simulink library "GearLibrary"  (R2017b)
settings: Solver=VariableStepAuto  StartTime=0.0  StopTime=10.0  RelTol=1e-3
undefined symbols (not defined in the file): c_LTset, DiscIntNeverNeededParam, g, Gear, magnitude, Strut, Tss, x1_LTset
libraries: GearLibrary x11, BaseLibrary x6, simulink x4, MathLibrary x2, vrlib x1
(part 2 of 2)

== system GearLibrary/Forces in Contact Point_Z2/If Action Subsystem1 ==
  v : Inport
  x : Inport  Port=2
  Action Port : ActionPort  InitializeStates=reset  ActionType=elseif
  " " : Saturate  UpperLimit=FOR_MaxDamp  LowerLimit=-FOR_MaxDamp
  Add : Sum
  Gain7 : Gain  Gain=d
  Gain8 : Gain  Gain=c
  Saturation : Saturate  UpperLimit=Compress_LengthMax*c  LowerLimit=-Compress_LengthMax*c
  Fz : Outport
  wires:
  v/1 -> Gain7/1  "x1dot"
  x/1 -> Gain8/1  "x1"
  Gain8/1 -> Saturation/1
  Add/1 -> Fz/1  "Fz1"
  Saturation/1 -> Add/2  "Fc"
  Gain7/1 -> " "/1
  " "/1 -> Add/1  "Fd"

== system GearLibrary/Forces in Contact Point_Z2/If Action Subsystem2 ==
  v : Inport
  x : Inport  Port=2
  Action Port : ActionPort  InitializeStates=reset  ActionType=else
  Add : Sum
  Constant : Constant  Value=Compress_LengthMax
  Constant1 : Constant  Value=Compress_LengthMax*c
  Fc2tox2 : Lookup_n-D  NumberOfTableDimensions=1  BreakpointsForDimension1=(linspace(0,Compress_LengthMax_Tire,30) * (9 * ct / Compress_LengthMax_Tire) + ct).*linspace(0,Compress_LengthMax_Tire,30)  Table=linspace(0,Compress_LengthMax_Tire,30)  InternalRulePriority=Speed  RndMeth=Simplest  InputSameDT=on
  Gain : Gain  Gain=-1
  Gain1 : Gain  Gain=-1
  Gain12 : Gain  Gain=dt
  Saturation : Saturate  UpperLimit=0  LowerLimit=-10*ct*Compress_LengthMax_Tire
  Sum : Sum  Inputs=|++
  Sum1 : Sum  Inputs=|+-
  x2toFc2 : Lookup_n-D  NumberOfTableDimensions=1  BreakpointsForDimension1=linspace(0,Compress_LengthMax_Tire,30)  Table=(linspace(0,Compress_LengthMax_Tire,30) * (9 * ct / Compress_LengthMax_Tire) + ct).*linspace(0,Compress_LengthMax_Tire,30)  InternalRulePriority=Speed  RndMeth=Simplest  InputSameDT=on
  Fz : Outport
  wires:
  x/1 -> Sum/1
  v/1 -> Gain12/1
  Sum/1 -> Sum1/1
  Constant/1 -> Sum/2
  x2toFc2/1 -> Gain1/1
  Gain12/1 -> Add/1  "Fdt"
  Saturation/1 -> Add/2  "Fct"
  Add/1 -> Fz/1  "Fz2"
  Constant1/1 -> Fc2tox2/1
  Sum1/1 -> Gain/1
  Gain/1 -> x2toFc2/1
  Gain1/1 -> Saturation/1
  Fc2tox2/1 -> Sum1/2

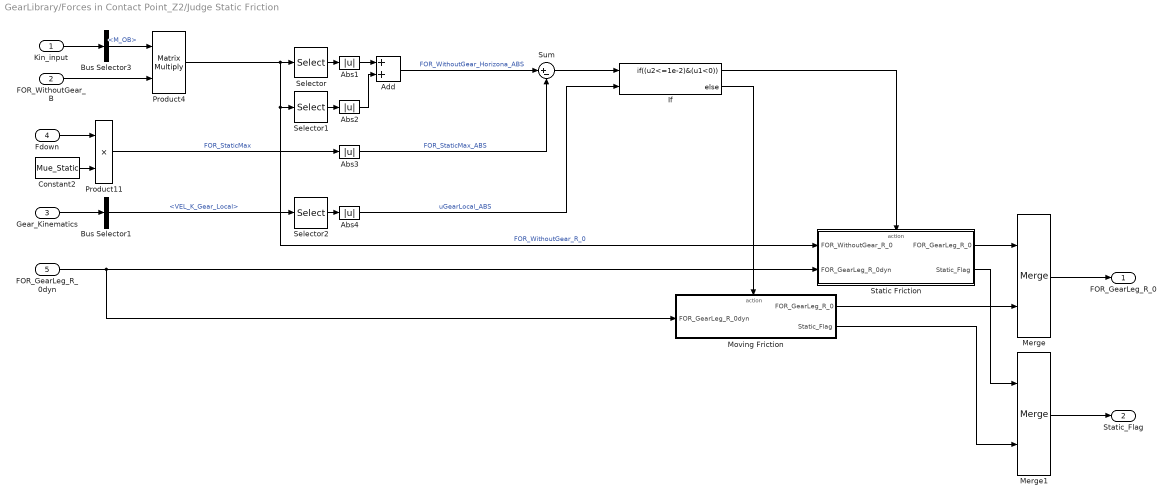
== system GearLibrary/Forces in Contact Point_Z2/Judge Static Friction ==
  Kin_input : Inport  OutDataTypeStr=Bus: Kin_input_BUS
  FOR_WithoutGear_B : Inport  Port=2  Unit=N  PortDimensions=[3 1]
  Gear_Kinematics : Inport  Port=3  OutDataTypeStr=Bus: GearKinematics_BUS
  Fdown : Inport  Port=4
  FOR_GearLeg_R_0dyn : Inport  Port=5
  Abs{1..4} (4 alike) : Abs
  Add : Sum
  Bus Selector1 : BusSelector  OutputSignals=VEL_K_Gear_Local
  Bus Selector3 : BusSelector  OutputSignals=M_OB
  Constant2 : Constant  Value=Mue_Static
  If : If  NumInputs=2  IfExpression=(u2<=1e-2)&(u1<0)
  Merge : Merge
  Merge1 : Merge
  Moving Friction : Subsystem  TreatAsAtomicUnit=on
  Product11 : Product
  Product4 : Product  Multiplication=Matrix(*)
  Selector : Selector  InputPortWidth=3  IndexOptions=Index vector (dialog)  Indices=[1]  OutputSizes=1
  Selector1 : Selector  InputPortWidth=3  IndexOptions=Index vector (dialog)  Indices=[2]  OutputSizes=1
  Selector2 : Selector  InputPortWidth=3  IndexOptions=Index vector (dialog)  Indices=[1]  OutputSizes=1
  "Static Friction " : Subsystem  TreatAsAtomicUnit=on
  Sum : Sum  Inputs=|+-
  FOR_GearLeg_R_0 : Outport  Unit=N  PortDimensions=[3,1]
  Static_Flag : Outport  Port=2  PortDimensions=[1]
  wires:
  "Static Friction "/2(Static_Flag) -> Merge1/1
  Merge1/1 -> Static_Flag/1
  Moving Friction/2(Static_Flag) -> Merge1/2
  Merge/1 -> FOR_GearLeg_R_0/1
  Moving Friction/1(FOR_GearLeg_R_0) -> Merge/2
  FOR_GearLeg_R_0dyn/1 -> Moving Friction/1(FOR_GearLeg_R_0dyn), "Static Friction "/2(FOR_GearLeg_R_0dyn)
  If/2 -> Moving Friction/Action
  "Static Friction "/1(FOR_GearLeg_R_0) -> Merge/1
  If/1 -> "Static Friction "/Action
  Abs4/1 -> If/2  "uGearLocal_ABS"
  Selector2/1 -> Abs4/1
  Bus Selector1/1 -> Selector2/1  "<VEL_K_Gear_Local>"
  Gear_Kinematics/1 -> Bus Selector1/1
  Sum/1 -> If/1
  Abs3/1 -> Sum/2  "FOR_StaticMax_ABS"
  Abs2/1 -> Add/2
  Selector1/1 -> Abs2/1
  Selector/1 -> Abs1/1
  Abs1/1 -> Add/1
  Add/1 -> Sum/1  "FOR_WithoutGear_Horizona_ABS"
  Product4/1 -> Selector/1, Selector1/1, "Static Friction "/1(FOR_WithoutGear_R_0)  "FOR_WithoutGear_R_0"
  FOR_WithoutGear_B/1 -> Product4/2
  Bus Selector3/1 -> Product4/1  "<M_OB>"
  Kin_input/1 -> Bus Selector3/1
  Product11/1 -> Abs3/1  "FOR_StaticMax"
  Constant2/1 -> Product11/2
  Fdown/1 -> Product11/1

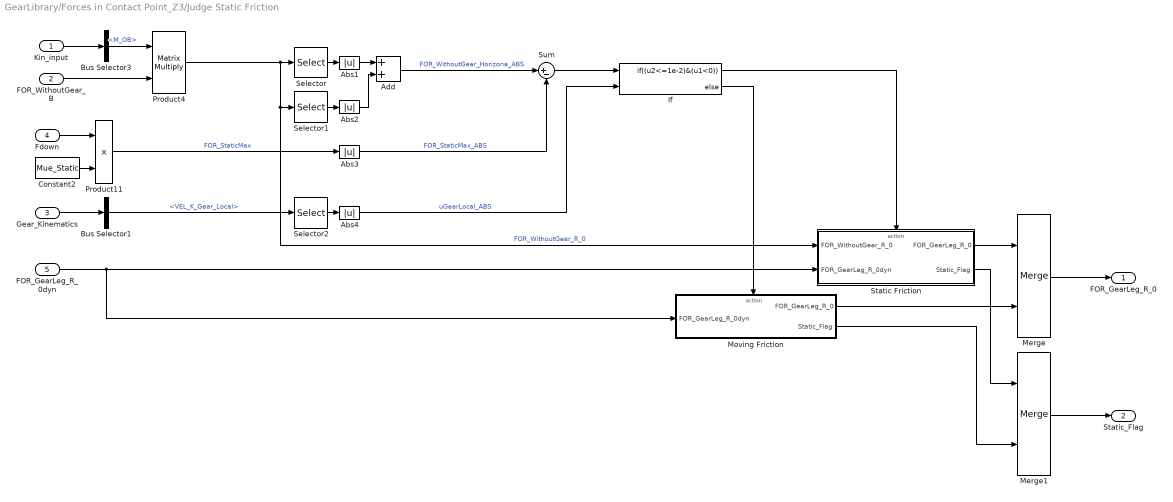
== system GearLibrary/Forces in Contact Point_Z3/Judge Static Friction ==
  Kin_input : Inport  OutDataTypeStr=Bus: Kin_input_BUS
  FOR_WithoutGear_B : Inport  Port=2  Unit=N  PortDimensions=[3 1]
  Gear_Kinematics : Inport  Port=3  OutDataTypeStr=Bus: GearKinematics_BUS
  Fdown : Inport  Port=4
  FOR_GearLeg_R_0dyn : Inport  Port=5
  Abs{1..4} (4 alike) : Abs
  Add : Sum
  Bus Selector1 : BusSelector  OutputSignals=VEL_K_Gear_Local
  Bus Selector3 : BusSelector  OutputSignals=M_OB
  Constant2 : Constant  Value=Mue_Static  SampleTime=Tss
  If : If  NumInputs=2  IfExpression=(u2<=1e-2)&(u1<0)
  Merge : Merge
  Merge1 : Merge
  Moving Friction : Subsystem  TreatAsAtomicUnit=on
  Product11 : Product
  Product4 : Product  Multiplication=Matrix(*)
  Selector : Selector  InputPortWidth=3  IndexOptions=Index vector (dialog)  Indices=[1]  OutputSizes=1
  Selector1 : Selector  InputPortWidth=3  IndexOptions=Index vector (dialog)  Indices=[2]  OutputSizes=1
  Selector2 : Selector  InputPortWidth=3  IndexOptions=Index vector (dialog)  Indices=[1]  OutputSizes=1
  "Static Friction " : Subsystem  TreatAsAtomicUnit=on
  Sum : Sum  Inputs=|+-
  FOR_GearLeg_R_0 : Outport  Unit=N  PortDimensions=[3,1]
  Static_Flag : Outport  Port=2  PortDimensions=[1]
  wires:
  "Static Friction "/2(Static_Flag) -> Merge1/1
  Merge1/1 -> Static_Flag/1
  Moving Friction/2(Static_Flag) -> Merge1/2
  Merge/1 -> FOR_GearLeg_R_0/1
  Moving Friction/1(FOR_GearLeg_R_0) -> Merge/2
  FOR_GearLeg_R_0dyn/1 -> Moving Friction/1(FOR_GearLeg_R_0dyn), "Static Friction "/2(FOR_GearLeg_R_0dyn)
  If/2 -> Moving Friction/Action
  "Static Friction "/1(FOR_GearLeg_R_0) -> Merge/1
  If/1 -> "Static Friction "/Action
  Abs4/1 -> If/2  "uGearLocal_ABS"
  Selector2/1 -> Abs4/1
  Bus Selector1/1 -> Selector2/1  "<VEL_K_Gear_Local>"
  Gear_Kinematics/1 -> Bus Selector1/1
  Sum/1 -> If/1
  Abs3/1 -> Sum/2  "FOR_StaticMax_ABS"
  Abs2/1 -> Add/2
  Selector1/1 -> Abs2/1
  Selector/1 -> Abs1/1
  Abs1/1 -> Add/1
  Add/1 -> Sum/1  "FOR_WithoutGear_Horizona_ABS"
  Product4/1 -> Selector/1, Selector1/1, "Static Friction "/1(FOR_WithoutGear_R_0)  "FOR_WithoutGear_R_0"
  FOR_WithoutGear_B/1 -> Product4/2
  Bus Selector3/1 -> Product4/1  "<M_OB>"
  Kin_input/1 -> Bus Selector3/1
  Product11/1 -> Abs3/1  "FOR_StaticMax"
  Constant2/1 -> Product11/2
  Fdown/1 -> Product11/1

== system GearLibrary/Gear Contact Point Dynamics/Calc VEL local lon//lat ==
  VEL_K_Gear_NED : Inport
  Tire Heading : Inport  Port=2  Unit=rad  PortDimensions=[1,1]
  Add : Sum
  Add1 : Sum
  Cos : Trigonometry  Operator=cos
  Cos1 : Trigonometry
  Cos2 : Trigonometry
  Cos3 : Trigonometry  Operator=cos
  Gain : Gain  Gain=-1
  Product{,1..3} (4 alike) : Product
  Vector Concatenate : Concatenate  NumInputs=3  Mode=Multidimensional array
  uB : Selector  InputPortWidth=3  IndexOptions=Index vector (dialog)  Indices=[1]  OutputSizes=1
  "uB " : Selector  InputPortWidth=3  IndexOptions=Index vector (dialog)  Indices=[1]  OutputSizes=1
  vB : Selector  InputPortWidth=3  IndexOptions=Index vector (dialog)  Indices=[2]  OutputSizes=1
  "vB " : Selector  InputPortWidth=3  IndexOptions=Index vector (dialog)  Indices=[2]  OutputSizes=1
  wB : Selector  InputPortWidth=3  IndexOptions=Index vector (dialog)  Indices=[3]  OutputSizes=1
  VEL_K_Gear_Local : Outport  Unit=m/s  PortDimensions=[3 1]
  wires:
  Tire Heading/1 -> Cos2/1, Cos3/1, Cos1/1, Cos/1
  VEL_K_Gear_NED/1 -> wB/1, "vB "/1, "uB "/1, vB/1, uB/1
  Cos/1 -> Product/1
  Product/1 -> Add/1
  uB/1 -> Product/2
  vB/1 -> Product1/2
  Cos1/1 -> Product1/1
  Product1/1 -> Add/2
  Add/1 -> Vector Concatenate/1
  Vector Concatenate/1 -> VEL_K_Gear_Local/1
  "uB "/1 -> Gain/1
  Gain/1 -> Product2/2
  Cos2/1 -> Product2/1
  "vB "/1 -> Product3/2
  Cos3/1 -> Product3/1
  Product3/1 -> Add1/2
  Product2/1 -> Add1/1
  Add1/1 -> Vector Concatenate/2
  wB/1 -> Vector Concatenate/3

== system GearLibrary/Gear Contact Point Dynamics/Norm ==
  V : Inport
  Math Function : Math  Operator=magnitude^2  SaturateOnIntegerOverflow=on
  Sqrt : Sqrt  SaturateOnIntegerOverflow=on
  Sum4 : Sum  Inputs=+
  ||V|| : Outport
  wires:
  Math Function/1 -> Sum4/1
  Sum4/1 -> Sqrt/1
  Sqrt/1 -> ||V||/1
  V/1 -> Math Function/1

== system GearLibrary/Gear Contact Point Dynamics/Subsystem ==
  Angle : Inport
  Trigonometric Function : Trigonometry  Operator=sincos
  Trigonometric Function1 : Trigonometry  Operator=atan2
  AngleWrap : Outport
  wires:
  Angle/1 -> Trigonometric Function/1
  Trigonometric Function/1 -> Trigonometric Function1/1
  Trigonometric Function/2 -> Trigonometric Function1/2
  Trigonometric Function1/1 -> AngleWrap/1

== system GearLibrary/Gear Contact Point Dynamics_WL1/Calc VEL local lon//lat ==
  VEL_K_Gear_NED : Inport
  Tire Heading : Inport  Port=2  Unit=rad  PortDimensions=[1,1]
  Add : Sum
  Add1 : Sum
  Cos : Trigonometry  Operator=cos
  Cos1 : Trigonometry
  Cos2 : Trigonometry
  Cos3 : Trigonometry  Operator=cos
  Gain : Gain  Gain=-1
  Product{,1..3} (4 alike) : Product
  Vector Concatenate : Concatenate  NumInputs=3  Mode=Multidimensional array
  uB : Selector  InputPortWidth=3  IndexOptions=Index vector (dialog)  Indices=[1]  OutputSizes=1
  "uB " : Selector  InputPortWidth=3  IndexOptions=Index vector (dialog)  Indices=[1]  OutputSizes=1
  vB : Selector  InputPortWidth=3  IndexOptions=Index vector (dialog)  Indices=[2]  OutputSizes=1
  "vB " : Selector  InputPortWidth=3  IndexOptions=Index vector (dialog)  Indices=[2]  OutputSizes=1
  wB : Selector  InputPortWidth=3  IndexOptions=Index vector (dialog)  Indices=[3]  OutputSizes=1
  VEL_K_Gear_Local : Outport  Unit=m/s  PortDimensions=[3 1]
  wires:
  wB/1 -> Vector Concatenate/3
  Add1/1 -> Vector Concatenate/2
  Product2/1 -> Add1/1
  Product3/1 -> Add1/2
  Cos3/1 -> Product3/1
  "vB "/1 -> Product3/2
  Cos2/1 -> Product2/1
  Gain/1 -> Product2/2
  "uB "/1 -> Gain/1
  Vector Concatenate/1 -> VEL_K_Gear_Local/1
  Add/1 -> Vector Concatenate/1
  Product1/1 -> Add/2
  Cos1/1 -> Product1/1
  vB/1 -> Product1/2
  uB/1 -> Product/2
  Product/1 -> Add/1
  Cos/1 -> Product/1
  VEL_K_Gear_NED/1 -> uB/1, vB/1, "uB "/1, "vB "/1, wB/1
  Tire Heading/1 -> Cos/1, Cos1/1, Cos3/1, Cos2/1

== system GearLibrary/Gear Contact Point Dynamics_WL1/Norm ==
  V : Inport
  Math Function : Math  Operator=magnitude^2  SaturateOnIntegerOverflow=on
  Sqrt : Sqrt  SaturateOnIntegerOverflow=on
  Sum4 : Sum  Inputs=+
  ||V|| : Outport
  wires:
  V/1 -> Math Function/1
  Sqrt/1 -> ||V||/1
  Sum4/1 -> Sqrt/1
  Math Function/1 -> Sum4/1

== system GearLibrary/Gear Contact Point Dynamics_WL1/Subsystem ==
  Angle : Inport
  Trigonometric Function : Trigonometry  Operator=sincos
  Trigonometric Function1 : Trigonometry  Operator=atan2
  AngleWrap : Outport
  wires:
  Trigonometric Function1/1 -> AngleWrap/1
  Trigonometric Function/2 -> Trigonometric Function1/2
  Trigonometric Function/1 -> Trigonometric Function1/1
  Angle/1 -> Trigonometric Function/1

== system GearLibrary/Forces in Contact Point/Judge Static Friction/Moving Friction ==
  FOR_GearLeg_R_0dyn : Inport
  Action Port : ActionPort  ActionType=else
  Constant : Constant  Value=0
  FOR_GearLeg_R_0 : Outport  Unit=N  PortDimensions=[3,1]
  Static_Flag : Outport  Port=2  PortDimensions=[1]
  wires:
  FOR_GearLeg_R_0dyn/1 -> FOR_GearLeg_R_0/1
  Constant/1 -> Static_Flag/1

== system GearLibrary/Forces in Contact Point/Judge Static Friction/Static Friction  ==
  FOR_WithoutGear_R_0 : Inport
  FOR_GearLeg_R_0dyn : Inport  Port=2
  Action Port : ActionPort  ActionType=then
  Constant : Constant
  Selector : Selector  InputPortWidth=3  IndexOptions=Index vector (dialog)  Indices=[1]  OutputSizes=1
  Selector1 : Selector  InputPortWidth=3  IndexOptions=Index vector (dialog)  Indices=[2]  OutputSizes=1
  Selector2 : Selector  InputPortWidth=3  IndexOptions=Index vector (dialog)  Indices=[3]  OutputSizes=1
  Vector Concatenate : Concatenate  NumInputs=3  Mode=Multidimensional array
  FOR_GearLeg_R_0 : Outport  Unit=N  PortDimensions=[3,1]
  Static_Flag : Outport  Port=2  PortDimensions=[1]
  wires:
  FOR_WithoutGear_R_0/1 -> Selector1/1, Selector/1
  FOR_GearLeg_R_0dyn/1 -> Selector2/1
  Selector/1 -> Vector Concatenate/1
  Selector1/1 -> Vector Concatenate/2
  Selector2/1 -> Vector Concatenate/3
  Vector Concatenate/1 -> FOR_GearLeg_R_0/1
  Constant/1 -> Static_Flag/1

== system GearLibrary/Forces in Contact Point_WL1/Judge Static Friction/Moving Friction ==
  FOR_GearLeg_R_0dyn : Inport
  Action Port : ActionPort
  Constant : Constant  Value=0
  FOR_GearLeg_R_0 : Outport  Unit=N  PortDimensions=[3,1]
  Static_Flag : Outport  Port=2  PortDimensions=[1]
  wires:
  FOR_GearLeg_R_0dyn/1 -> FOR_GearLeg_R_0/1
  Constant/1 -> Static_Flag/1

== system GearLibrary/Forces in Contact Point_WL1/Judge Static Friction/Static Friction  ==
  FOR_WithoutGear_R_0 : Inport
  FOR_GearLeg_R_0dyn : Inport  Port=2
  Action Port : ActionPort
  Constant : Constant
  Selector : Selector  InputPortWidth=3  IndexOptions=Index vector (dialog)  Indices=[1]  OutputSizes=1
  Selector1 : Selector  InputPortWidth=3  IndexOptions=Index vector (dialog)  Indices=[2]  OutputSizes=1
  Selector2 : Selector  InputPortWidth=3  IndexOptions=Index vector (dialog)  Indices=[3]  OutputSizes=1
  Vector Concatenate : Concatenate  NumInputs=3  Mode=Multidimensional array
  FOR_GearLeg_R_0 : Outport  Unit=N  PortDimensions=[3,1]
  Static_Flag : Outport  Port=2  PortDimensions=[1]
  wires:
  FOR_WithoutGear_R_0/1 -> Selector1/1, Selector/1
  FOR_GearLeg_R_0dyn/1 -> Selector2/1
  Selector/1 -> Vector Concatenate/1
  Selector1/1 -> Vector Concatenate/2
  Selector2/1 -> Vector Concatenate/3
  Vector Concatenate/1 -> FOR_GearLeg_R_0/1
  Constant/1 -> Static_Flag/1

== system GearLibrary/Forces in Contact Point_Z1/Judge Static Friction/Moving Friction ==
  FOR_GearLeg_R_0dyn : Inport
  Action Port : ActionPort
  Constant : Constant  Value=0
  FOR_GearLeg_R_0 : Outport  Unit=N  PortDimensions=[3,1]
  Static_Flag : Outport  Port=2  PortDimensions=[1]
  wires:
  FOR_GearLeg_R_0dyn/1 -> FOR_GearLeg_R_0/1
  Constant/1 -> Static_Flag/1

== system GearLibrary/Forces in Contact Point_Z1/Judge Static Friction/Static Friction  ==
  FOR_WithoutGear_R_0 : Inport
  FOR_GearLeg_R_0dyn : Inport  Port=2
  Action Port : ActionPort
  Constant : Constant
  Selector : Selector  InputPortWidth=3  IndexOptions=Index vector (dialog)  Indices=[1]  OutputSizes=1
  Selector1 : Selector  InputPortWidth=3  IndexOptions=Index vector (dialog)  Indices=[2]  OutputSizes=1
  Selector2 : Selector  InputPortWidth=3  IndexOptions=Index vector (dialog)  Indices=[3]  OutputSizes=1
  Vector Concatenate : Concatenate  NumInputs=3  Mode=Multidimensional array
  FOR_GearLeg_R_0 : Outport  Unit=N  PortDimensions=[3,1]
  Static_Flag : Outport  Port=2  PortDimensions=[1]
  wires:
  FOR_WithoutGear_R_0/1 -> Selector1/1, Selector/1
  FOR_GearLeg_R_0dyn/1 -> Selector2/1
  Selector/1 -> Vector Concatenate/1
  Selector1/1 -> Vector Concatenate/2
  Selector2/1 -> Vector Concatenate/3
  Vector Concatenate/1 -> FOR_GearLeg_R_0/1
  Constant/1 -> Static_Flag/1

== system GearLibrary/Forces in Contact Point_Z2/Judge Static Friction/Moving Friction ==
  FOR_GearLeg_R_0dyn : Inport
  Action Port : ActionPort
  Constant : Constant  Value=0
  FOR_GearLeg_R_0 : Outport  Unit=N  PortDimensions=[3,1]
  Static_Flag : Outport  Port=2  PortDimensions=[1]
  wires:
  Constant/1 -> Static_Flag/1
  FOR_GearLeg_R_0dyn/1 -> FOR_GearLeg_R_0/1

== system GearLibrary/Forces in Contact Point_Z2/Judge Static Friction/Static Friction  ==
  FOR_WithoutGear_R_0 : Inport
  FOR_GearLeg_R_0dyn : Inport  Port=2
  Action Port : ActionPort
  Constant : Constant
  Selector : Selector  InputPortWidth=3  IndexOptions=Index vector (dialog)  Indices=[1]  OutputSizes=1
  Selector1 : Selector  InputPortWidth=3  IndexOptions=Index vector (dialog)  Indices=[2]  OutputSizes=1
  Selector2 : Selector  InputPortWidth=3  IndexOptions=Index vector (dialog)  Indices=[3]  OutputSizes=1
  Vector Concatenate : Concatenate  NumInputs=3  Mode=Multidimensional array
  FOR_GearLeg_R_0 : Outport  Unit=N  PortDimensions=[3,1]
  Static_Flag : Outport  Port=2  PortDimensions=[1]
  wires:
  Constant/1 -> Static_Flag/1
  Vector Concatenate/1 -> FOR_GearLeg_R_0/1
  Selector2/1 -> Vector Concatenate/3
  Selector1/1 -> Vector Concatenate/2
  Selector/1 -> Vector Concatenate/1
  FOR_GearLeg_R_0dyn/1 -> Selector2/1
  FOR_WithoutGear_R_0/1 -> Selector/1, Selector1/1

== system GearLibrary/Forces in Contact Point_Z3/Judge Static Friction/Moving Friction ==
  FOR_GearLeg_R_0dyn : Inport
  Action Port : ActionPort
  Constant : Constant  Value=0
  FOR_GearLeg_R_0 : Outport  Unit=N  PortDimensions=[3,1]
  Static_Flag : Outport  Port=2  PortDimensions=[1]
  wires:
  Constant/1 -> Static_Flag/1
  FOR_GearLeg_R_0dyn/1 -> FOR_GearLeg_R_0/1

== system GearLibrary/Forces in Contact Point_Z3/Judge Static Friction/Static Friction  ==
  FOR_WithoutGear_R_0 : Inport
  FOR_GearLeg_R_0dyn : Inport  Port=2
  Action Port : ActionPort
  Constant : Constant
  Selector : Selector  InputPortWidth=3  IndexOptions=Index vector (dialog)  Indices=[1]  OutputSizes=1
  Selector1 : Selector  InputPortWidth=3  IndexOptions=Index vector (dialog)  Indices=[2]  OutputSizes=1
  Selector2 : Selector  InputPortWidth=3  IndexOptions=Index vector (dialog)  Indices=[3]  OutputSizes=1
  Vector Concatenate : Concatenate  NumInputs=3  Mode=Multidimensional array
  FOR_GearLeg_R_0 : Outport  Unit=N  PortDimensions=[3,1]
  Static_Flag : Outport  Port=2  PortDimensions=[1]
  wires:
  Constant/1 -> Static_Flag/1
  Vector Concatenate/1 -> FOR_GearLeg_R_0/1
  Selector2/1 -> Vector Concatenate/3
  Selector1/1 -> Vector Concatenate/2
  Selector/1 -> Vector Concatenate/1
  FOR_GearLeg_R_0dyn/1 -> Selector2/1
  FOR_WithoutGear_R_0/1 -> Selector/1, Selector1/1
